simulink model "model_polozenie"  (R2014a)
settings: Solver=ode4  StartTime=0.0  StopTime=10  FixedStep=0.01  RelTol=1e-3
settings Model: Creator=Cula  LastModifiedBy=Praca

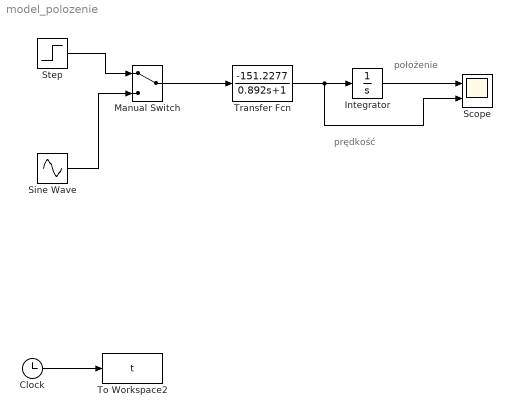
== system model_polozenie ==
  note: prędkość
  note: położenie
  Clock : Clock
  Integrator : Integrator
  Manual Switch : ManualSwitch
  Scope : Scope  NumInputPorts=2
      settings: YMin=-5~-5  YMax=5~5
  Sine Wave : Sin  Amplitude=100  SampleTime=0
  Step : Step  Time=2  SampleTime=0
  To Workspace2 : ToWorkspace  VariableName=t  SaveFormat=Timeseries  SampleTime=-1
  Transfer Fcn : TransferFcn  Numerator=[-151.2277]  Denominator=[0.892 1]
  wires:
  Step/1 -> Manual Switch/1
  Sine Wave/1 -> Manual Switch/2
  Manual Switch/1 -> Transfer Fcn/1
  Clock/1 -> To Workspace2/1
  Transfer Fcn/1 -> Scope/2, Integrator/1
  Integrator/1 -> Scope/1
